simulink model "PD_controller"  (R2018a)
settings: Solver=VariableStepAuto  StartTime=0.0  StopTime=200  RelTol=1e-3
settings Model: Creator=mjb15180  LastModifiedBy=mjb15180

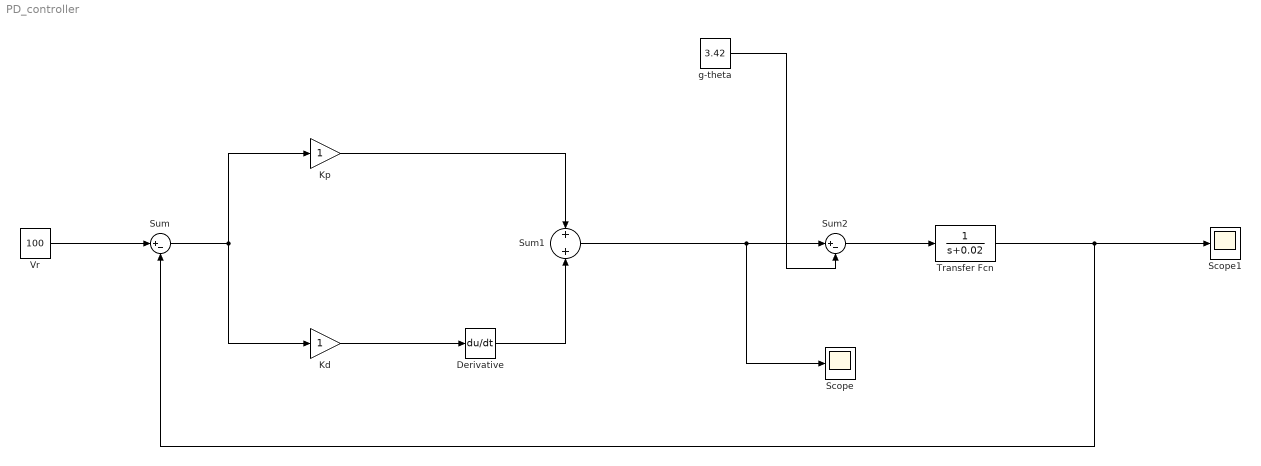
== system PD_controller ==
  Derivative : Derivative  CoefficientInTFapproximation=1
  Kd : Gain
  Kp : Gain
  Scope : Scope
  Scope1 : Scope
  Sum : Sum  Inputs=|+-
  Sum1 : Sum
  Sum2 : Sum  Inputs=|+-
  Transfer Fcn : TransferFcn  Denominator=[1 0.02]
  Vr : Constant  Value=100
  g-theta : Constant  Value=3.42
  wires:
  Sum2/1 -> Transfer Fcn/1
  Transfer Fcn/1 -> Sum/2, Scope1/1
  Kp/1 -> Sum1/1
  Sum1/1 -> Scope/1, Sum2/1
  g-theta/1 -> Sum2/2
  Kd/1 -> Derivative/1
  Sum/1 -> Kd/1, Kp/1
  Vr/1 -> Sum/1
  Derivative/1 -> Sum1/2
